simulink model "CIC_decimator_HDL_model"  (R2018b)
settings: Solver=FixedStepAuto  StartTime=0.0  StopTime=10  RelTol=1e-3  EnableMultiTasking=on
values from neighbouring files (symbols this model uses):
  Fs = 2e6    (= 2000000)    [CIC_decimation_with_comp.m]
  ftest1 = 1e3    (= 1000)    [CIC_decimation_with_comp.m]
  ftest2 = 4e3    (= 4000)    [CIC_decimation_with_comp.m]
  ftest3 = 12e3    (= 12000)    [CIC_decimation_with_comp.m]
  hz = int32(round(h * power(2, B - 1) - 1))    [CIC_decimation_with_comp.m]
  R = 125    [CIC_decimation_with_comp.m]
  scaling_numerator = 11    [CIC_decimation_with_comp.m]
undefined symbols (not defined in the file or in its folder): DiscIntNeverNeededParam
libraries: hdlsllib x28, dspsrcs4 x3, simulink x2, commchan3 x1
settings Model: Creator=MrGoshak  LastModifiedBy=MrGoshak
settings HardwareCC: ProdBitPerPointer=32  ProdBitPerSizeT=32  ProdBitPerPtrDiffT=32  ProdLargestAtomicFloat=None  ProdIntDivRoundTo=Undefined  ProdEndianess=Unspecified  ProdWordSize=32  ProdHWDeviceType=ASIC/FPGA->ASIC/FPGA  TargetBitPerPointer=64  TargetBitPerSizeT=64  TargetBitPerPtrDiffT=64  TargetLongLongMode=on  TargetIntDivRoundTo=Zero  TargetEndianess=LittleEndian  TargetWordSize=64  TargetHWDeviceType=Custom Processor->MATLAB Host Computer  ProdEqTarget=off

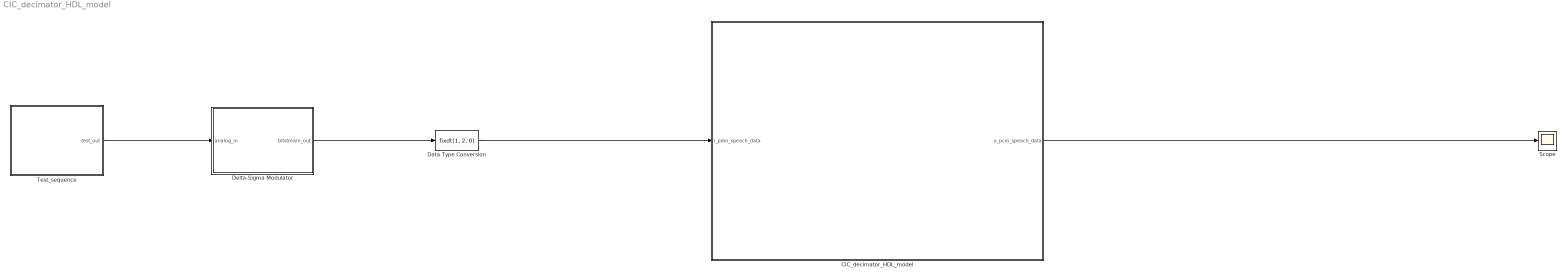
== system CIC_decimator_HDL_model ==
  CIC_decimator_HDL_model : Subsystem
  Data Type Conversion : DataTypeConversion  OutDataTypeStr=fixdt(1, 2, 0)
  "Delta-Sigma Modulator " : Subsystem
  Scope : Scope
  "Test_sequence " : Subsystem
  wires:
  "Test_sequence "/1(test_out) -> "Delta-Sigma Modulator "/1(analog_in)
  "Delta-Sigma Modulator "/1(bitstream_out) -> Data Type Conversion/1
  Data Type Conversion/1 -> CIC_decimator_HDL_model/1(i_pdm_speach_data)
  CIC_decimator_HDL_model/1(o_pcm_speach_data) -> Scope/1

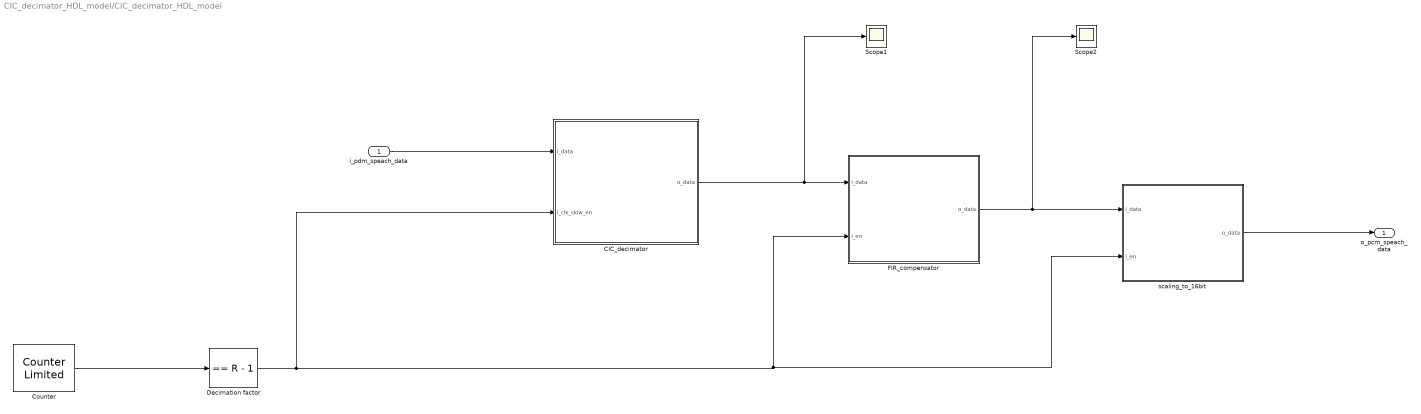
== system CIC_decimator_HDL_model/CIC_decimator_HDL_model ==
  i_pdm_speach_data : Inport
  CIC_decimator : Subsystem  Tag=FilterWizardSubSystem
      settings: ErrorFcn=dspFilterRealizedInBasicElemsAlgLoopErrFcnCallback
  "Counter " : simulink/Sources/Counter Limited  uplimit=R - 1  tsamp=1/Fs
  Decimation factor : simulink/Logic and Bit Operations/Compare To Constant  relop===  const=R - 1  OutDataTypeStr=boolean
  FIR_compensator : Subsystem  Tag=FilterWizardSubSystem
      settings: ErrorFcn=dspFilterRealizedInBasicElemsAlgLoopErrFcnCallback
  Scope1 : Scope
  Scope2 : Scope
  scaling_to_16bit : Subsystem
  o_pcm_speach_data : Outport
  wires:
  FIR_compensator/1(o_data) -> Scope2/1, scaling_to_16bit/1(i_data)
  i_pdm_speach_data/1 -> CIC_decimator/1(i_data)
  CIC_decimator/1(o_data) -> Scope1/1, FIR_compensator/1(i_data)
  scaling_to_16bit/1(o_data) -> o_pcm_speach_data/1
  Decimation factor/1 -> CIC_decimator/2(i_clk_slow_en), FIR_compensator/2(i_en), scaling_to_16bit/2(i_en)
  "Counter "/1 -> Decimation factor/1

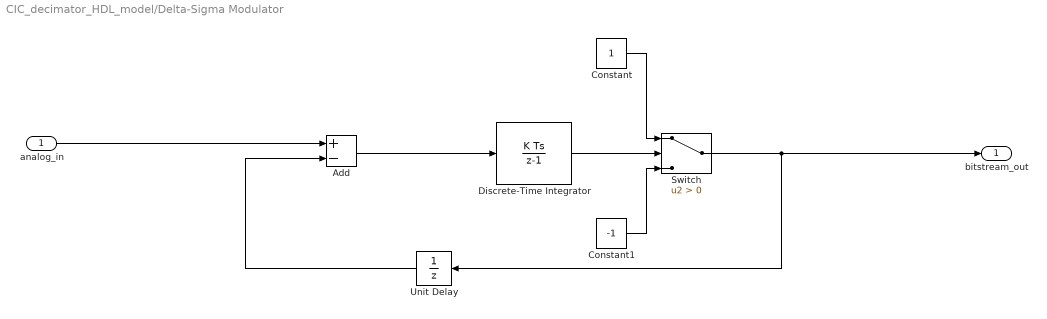
== system CIC_decimator_HDL_model/Delta-Sigma Modulator  ==
  analog_in : Inport
  Add : Sum  Inputs=+-
  Constant : Constant
  Constant1 : Constant  Value=-1
  Discrete-Time Integrator : DiscreteIntegrator  SampleTime=-1  ICPrevOutput=DiscIntNeverNeededParam  ICPrevScaledInput=DiscIntNeverNeededParam
  Switch : Switch  Criteria=u2 > Threshold
  Unit Delay : UnitDelay  SampleTime=-1
  bitstream_out : Outport
  wires:
  Unit Delay/1 -> Add/2
  Discrete-Time Integrator/1 -> Switch/2
  analog_in/1 -> Add/1
  Add/1 -> Discrete-Time Integrator/1
  Constant1/1 -> Switch/3
  Constant/1 -> Switch/1
  Switch/1 -> bitstream_out/1, Unit Delay/1

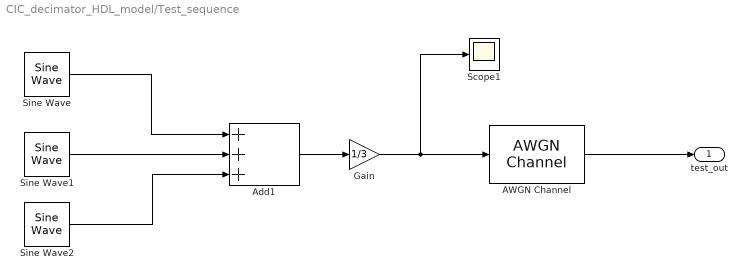
== system CIC_decimator_HDL_model/Test_sequence  ==
  AWGN Channel : commchan3/AWGN Channel  InputProcessing=Columns as channels (frame based)  seed=67  noiseMode="Signal to noise ratio  (SNR)"  EbNodB=10  EsNodB=10  SNRdB=40  bitsPerSym=1  Ps=1  Tsym=1  variance=1
  Add1 : Sum  Inputs=+++
  Gain : Gain  Gain=1/3
  Scope1 : Scope
  Sine Wave : dspsrcs4/Sine Wave  Amplitude=1  Frequency=ftest1  Phase=0  SampleMode=Discrete  OutComplex=Real  CompMethod=Trigonometric fcn  TableSize=Speed  SampleTime=1/Fs  SamplesPerFrame=1  ResetState=Restart at time zero  OutputFrames=off  dataType=double  wordLen=16  udDataType=sfix(16)  fracBitsMode=User-defined  numFracBits=0  OutDataTypeStr=double  LastOutDataTypeStr=double
  Sine Wave1 : dspsrcs4/Sine Wave  Amplitude=1  Frequency=ftest2  Phase=0  SampleMode=Discrete  OutComplex=Real  CompMethod=Trigonometric fcn  TableSize=Speed  SampleTime=1/Fs  SamplesPerFrame=1  ResetState=Restart at time zero  OutputFrames=off  dataType=double  wordLen=16  udDataType=sfix(16)  fracBitsMode=Best precision  numFracBits=15  OutDataTypeStr=double  LastOutDataTypeStr=double
  Sine Wave2 : dspsrcs4/Sine Wave  Amplitude=1  Frequency=ftest3  Phase=0  SampleMode=Discrete  OutComplex=Real  CompMethod=Trigonometric fcn  TableSize=Speed  SampleTime=1/Fs  SamplesPerFrame=1  ResetState=Restart at time zero  OutputFrames=off  dataType=double  wordLen=16  udDataType=sfix(16)  fracBitsMode=Best precision  numFracBits=15  OutDataTypeStr=double  LastOutDataTypeStr=double
  test_out : Outport
  wires:
  Sine Wave2/1 -> Add1/3
  Sine Wave/1 -> Add1/1
  Add1/1 -> Gain/1
  Gain/1 -> AWGN Channel/1, Scope1/1
  Sine Wave1/1 -> Add1/2
  AWGN Channel/1 -> test_out/1

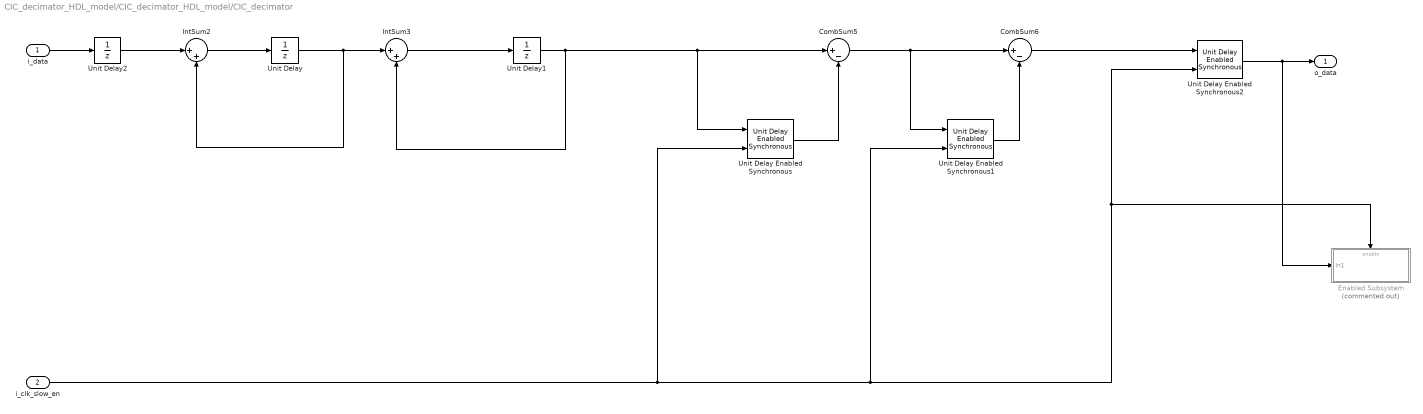
== system CIC_decimator_HDL_model/CIC_decimator_HDL_model/CIC_decimator ==
  i_data : Inport  SampleTime=1/Fs
  i_clk_slow_en : Inport  Port=2
  CombSum5 : Sum  Inputs=|+-  OutDataTypeStr=CIC_data_type
  CombSum6 : Sum  Inputs=|+-  OutDataTypeStr=CIC_data_type
  Enabled Subsystem : Subsystem  Commented=on  TreatAsAtomicUnit=on
  IntSum2 : Sum  Inputs=|++  OutDataTypeStr=CIC_data_type
  IntSum3 : Sum  Inputs=|++  OutDataTypeStr=CIC_data_type
  Unit Delay : UnitDelay  SampleTime=-1
  Unit Delay Enabled Synchronous : hdlsllib/Discrete/Unit Delay Enabled Synchronous  InitialCondition=0.0  SampleTime=-1
      settings: SourceProductName=HDL Coder  SourceProductBaseCode=HD
  Unit Delay Enabled Synchronous1 : hdlsllib/Discrete/Unit Delay Enabled Synchronous  InitialCondition=0.0  SampleTime=-1
      settings: SourceProductName=HDL Coder  SourceProductBaseCode=HD
  Unit Delay Enabled Synchronous2 : hdlsllib/Discrete/Unit Delay Enabled Synchronous  InitialCondition=0.0  SampleTime=-1
      settings: SourceProductName=HDL Coder  SourceProductBaseCode=HD
  Unit Delay1 : UnitDelay  SampleTime=-1
  Unit Delay2 : UnitDelay  SampleTime=-1
  o_data : Outport
  wires:
  i_data/1 -> Unit Delay2/1
  Unit Delay/1 -> IntSum2/2, IntSum3/1
  IntSum3/1 -> Unit Delay1/1
  CombSum5/1 -> Unit Delay Enabled Synchronous1/1, CombSum6/1
  Unit Delay Enabled Synchronous/1 -> CombSum5/2
  Unit Delay Enabled Synchronous1/1 -> CombSum6/2
  CombSum6/1 -> Unit Delay Enabled Synchronous2/1
  Unit Delay Enabled Synchronous2/1 -> Enabled Subsystem/1(In1), o_data/1
  IntSum2/1 -> Unit Delay/1
  Unit Delay1/1 -> IntSum3/2, Unit Delay Enabled Synchronous/1, CombSum5/1
  i_clk_slow_en/1 -> Unit Delay Enabled Synchronous1/2, Enabled Subsystem/Enable, Unit Delay Enabled Synchronous2/2, Unit Delay Enabled Synchronous/2
  Unit Delay2/1 -> IntSum2/1

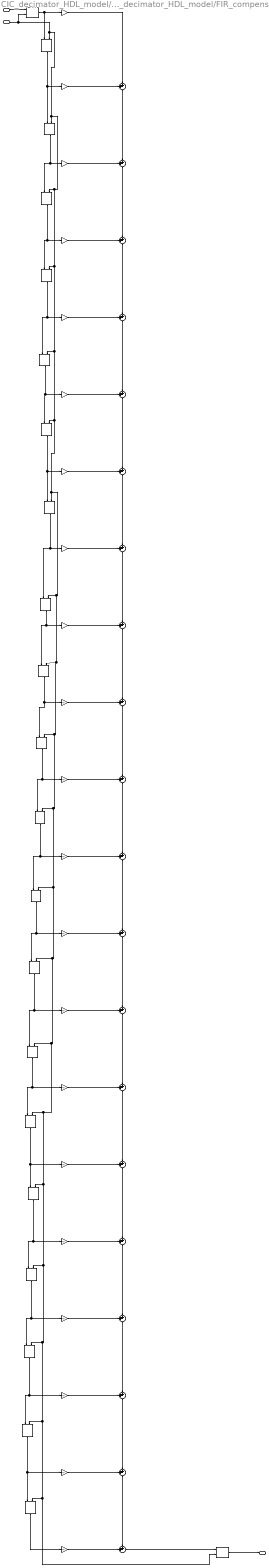
== system CIC_decimator_HDL_model/CIC_decimator_HDL_model/FIR_compensator ==
  i_data : Inport
  i_en : Inport  Port=2
  BodyLSum{2..21} (20 alike) : Sum  Inputs=++|  AccumDataTypeStr=FIR_product_data_type  OutDataTypeStr=FIR_product_data_type  SaturateOnIntegerOverflow=on
  Unit Delay Enabled Synchronous{,1..21} (22 alike) : hdlsllib/Discrete/Unit Delay Enabled Synchronous  InitialCondition=0.0  SampleTime=-1
      settings: SourceProductName=HDL Coder  SourceProductBaseCode=HD
  b(1) : Gain  Gain=hz(1)  ParamDataTypeStr=FIR_coeffs_data_type  OutDataTypeStr=FIR_product_data_type  SaturateOnIntegerOverflow=on
  b(10) : Gain  Gain=hz(10)  ParamDataTypeStr=FIR_coeffs_data_type  OutDataTypeStr=FIR_product_data_type  SaturateOnIntegerOverflow=on
  b(11) : Gain  Gain=hz(11)  ParamDataTypeStr=FIR_coeffs_data_type  OutDataTypeStr=FIR_product_data_type  SaturateOnIntegerOverflow=on
  b(12) : Gain  Gain=hz(12)  ParamDataTypeStr=FIR_coeffs_data_type  OutDataTypeStr=FIR_product_data_type  SaturateOnIntegerOverflow=on
  b(13) : Gain  Gain=hz(13)  ParamDataTypeStr=FIR_coeffs_data_type  OutDataTypeStr=FIR_product_data_type  SaturateOnIntegerOverflow=on
  b(14) : Gain  Gain=hz(14)  ParamDataTypeStr=FIR_coeffs_data_type  OutDataTypeStr=FIR_product_data_type  SaturateOnIntegerOverflow=on
  b(15) : Gain  Gain=hz(15)  ParamDataTypeStr=FIR_coeffs_data_type  OutDataTypeStr=FIR_product_data_type  SaturateOnIntegerOverflow=on
  b(16) : Gain  Gain=hz(16)  ParamDataTypeStr=FIR_coeffs_data_type  OutDataTypeStr=FIR_product_data_type  SaturateOnIntegerOverflow=on
  b(17) : Gain  Gain=hz(17)  ParamDataTypeStr=FIR_coeffs_data_type  OutDataTypeStr=FIR_product_data_type  SaturateOnIntegerOverflow=on
  b(18) : Gain  Gain=hz(18)  ParamDataTypeStr=FIR_coeffs_data_type  OutDataTypeStr=FIR_product_data_type  SaturateOnIntegerOverflow=on
  b(19) : Gain  Gain=hz(19)  ParamDataTypeStr=FIR_coeffs_data_type  OutDataTypeStr=FIR_product_data_type  SaturateOnIntegerOverflow=on
  b(2) : Gain  Gain=hz(2)  ParamDataTypeStr=FIR_coeffs_data_type  OutDataTypeStr=FIR_product_data_type  SaturateOnIntegerOverflow=on
  b(20) : Gain  Gain=hz(20)  ParamDataTypeStr=FIR_coeffs_data_type  OutDataTypeStr=FIR_product_data_type  SaturateOnIntegerOverflow=on
  b(21) : Gain  Gain=hz(21)  ParamDataTypeStr=FIR_coeffs_data_type  OutDataTypeStr=FIR_product_data_type  SaturateOnIntegerOverflow=on
  b(3) : Gain  Gain=hz(3)  ParamDataTypeStr=FIR_coeffs_data_type  OutDataTypeStr=FIR_product_data_type  SaturateOnIntegerOverflow=on
  b(4) : Gain  Gain=hz(4)  ParamDataTypeStr=FIR_coeffs_data_type  OutDataTypeStr=FIR_product_data_type  SaturateOnIntegerOverflow=on
  b(5) : Gain  Gain=hz(5)  ParamDataTypeStr=FIR_coeffs_data_type  OutDataTypeStr=FIR_product_data_type  SaturateOnIntegerOverflow=on
  b(6) : Gain  Gain=hz(6)  ParamDataTypeStr=FIR_coeffs_data_type  OutDataTypeStr=FIR_product_data_type  SaturateOnIntegerOverflow=on
  b(7) : Gain  Gain=hz(7)  ParamDataTypeStr=FIR_coeffs_data_type  OutDataTypeStr=FIR_product_data_type  SaturateOnIntegerOverflow=on
  b(8) : Gain  Gain=hz(8)  ParamDataTypeStr=FIR_coeffs_data_type  OutDataTypeStr=FIR_product_data_type  SaturateOnIntegerOverflow=on
  b(9) : Gain  Gain=hz(9)  ParamDataTypeStr=FIR_coeffs_data_type  OutDataTypeStr=FIR_product_data_type  SaturateOnIntegerOverflow=on
  o_data : Outport
  wires:
  b(1)/1 -> BodyLSum2/2
  Unit Delay Enabled Synchronous/1 -> Unit Delay Enabled Synchronous1/1, b(2)/1
  b(2)/1 -> BodyLSum2/1
  BodyLSum2/1 -> BodyLSum3/2
  b(3)/1 -> BodyLSum3/1
  BodyLSum3/1 -> BodyLSum4/2
  Unit Delay Enabled Synchronous2/1 -> Unit Delay Enabled Synchronous3/1, b(4)/1
  b(4)/1 -> BodyLSum4/1
  BodyLSum4/1 -> BodyLSum5/2
  Unit Delay Enabled Synchronous3/1 -> b(5)/1, Unit Delay Enabled Synchronous4/1
  b(5)/1 -> BodyLSum5/1
  BodyLSum5/1 -> BodyLSum6/2
  b(6)/1 -> BodyLSum6/1
  BodyLSum6/1 -> BodyLSum7/2
  Unit Delay Enabled Synchronous5/1 -> b(7)/1, Unit Delay Enabled Synchronous6/1
  b(7)/1 -> BodyLSum7/1
  BodyLSum7/1 -> BodyLSum8/2
  b(8)/1 -> BodyLSum8/1
  BodyLSum8/1 -> BodyLSum9/2
  b(9)/1 -> BodyLSum9/1
  BodyLSum9/1 -> BodyLSum10/2
  b(10)/1 -> BodyLSum10/1
  BodyLSum10/1 -> BodyLSum11/2
  b(11)/1 -> BodyLSum11/1
  BodyLSum11/1 -> BodyLSum12/2
  b(12)/1 -> BodyLSum12/1
  BodyLSum12/1 -> BodyLSum13/2
  b(13)/1 -> BodyLSum13/1
  BodyLSum13/1 -> BodyLSum14/2
  b(14)/1 -> BodyLSum14/1
  BodyLSum14/1 -> BodyLSum15/2
  b(15)/1 -> BodyLSum15/1
  BodyLSum15/1 -> BodyLSum16/2
  b(16)/1 -> BodyLSum16/1
  BodyLSum16/1 -> BodyLSum17/2
  b(17)/1 -> BodyLSum17/1
  BodyLSum17/1 -> BodyLSum18/2
  b(18)/1 -> BodyLSum18/1
  BodyLSum18/1 -> BodyLSum19/2
  b(19)/1 -> BodyLSum19/1
  BodyLSum19/1 -> BodyLSum20/2
  b(20)/1 -> BodyLSum20/1
  BodyLSum20/1 -> BodyLSum21/1
  b(21)/1 -> BodyLSum21/2
  Unit Delay Enabled Synchronous1/1 -> Unit Delay Enabled Synchronous2/1, b(3)/1
  Unit Delay Enabled Synchronous4/1 -> b(6)/1, Unit Delay Enabled Synchronous5/1
  Unit Delay Enabled Synchronous6/1 -> Unit Delay Enabled Synchronous7/1, b(8)/1
  Unit Delay Enabled Synchronous7/1 -> Unit Delay Enabled Synchronous8/1, b(9)/1
  Unit Delay Enabled Synchronous8/1 -> Unit Delay Enabled Synchronous9/1, b(10)/1
  Unit Delay Enabled Synchronous9/1 -> Unit Delay Enabled Synchronous10/1, b(11)/1
  Unit Delay Enabled Synchronous10/1 -> Unit Delay Enabled Synchronous11/1, b(12)/1
  Unit Delay Enabled Synchronous11/1 -> Unit Delay Enabled Synchronous12/1, b(13)/1
  Unit Delay Enabled Synchronous12/1 -> Unit Delay Enabled Synchronous13/1, b(14)/1
  Unit Delay Enabled Synchronous13/1 -> Unit Delay Enabled Synchronous14/1, b(15)/1
  Unit Delay Enabled Synchronous14/1 -> b(16)/1, Unit Delay Enabled Synchronous15/1
  Unit Delay Enabled Synchronous15/1 -> Unit Delay Enabled Synchronous16/1, b(17)/1
  Unit Delay Enabled Synchronous16/1 -> Unit Delay Enabled Synchronous17/1, b(18)/1
  Unit Delay Enabled Synchronous17/1 -> b(19)/1, Unit Delay Enabled Synchronous18/1
  Unit Delay Enabled Synchronous18/1 -> b(20)/1, Unit Delay Enabled Synchronous19/1
  Unit Delay Enabled Synchronous19/1 -> b(21)/1
  Unit Delay Enabled Synchronous20/1 -> o_data/1
  i_data/1 -> Unit Delay Enabled Synchronous21/1
  Unit Delay Enabled Synchronous21/1 -> Unit Delay Enabled Synchronous/1, b(1)/1
  i_en/1 -> Unit Delay Enabled Synchronous20/2, Unit Delay Enabled Synchronous19/2, Unit Delay Enabled Synchronous18/2, Unit Delay Enabled Synchronous17/2, Unit Delay Enabled Synchronous16/2, Unit Delay Enabled Synchronous15/2, Unit Delay Enabled Synchronous14/2, Unit Delay Enabled Synchronous13/2, Unit Delay Enabled Synchronous12/2, Unit Delay Enabled Synchronous11/2, Unit Delay Enabled Synchronous10/2, Unit Delay Enabled Synchronous9/2, Unit Delay Enabled Synchronous8/2, Unit Delay Enabled Synchronous7/2, Unit Delay Enabled Synchronous6/2, Unit Delay Enabled Synchronous5/2, Unit Delay Enabled Synchronous4/2, Unit Delay Enabled Synchronous3/2, Unit Delay Enabled Synchronous2/2, Unit Delay Enabled Synchronous1/2, Unit Delay Enabled Synchronous/2, Unit Delay Enabled Synchronous21/2
  BodyLSum21/1 -> Unit Delay Enabled Synchronous20/1

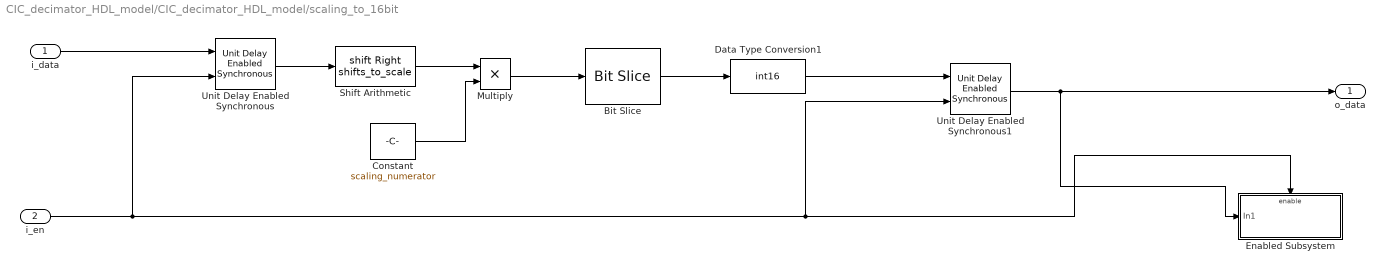
== system CIC_decimator_HDL_model/CIC_decimator_HDL_model/scaling_to_16bit ==
  i_data : Inport
  i_en : Inport  Port=2
  Bit Slice : hdlsllib/Logic and Bit Operations/Bit Slice  lidx=30  ridx=15
  Constant : Constant  Value=scaling_numerator  OutDataTypeStr=uint8  SampleTime=1/Fs
  Data Type Conversion1 : DataTypeConversion  OutDataTypeStr=int16
  Enabled Subsystem : Subsystem  TreatAsAtomicUnit=on
  Multiply : Product  OutDataTypeStr=fixdt(1,31,0)  SaturateOnIntegerOverflow=on
  Shift Arithmetic : ArithShift  BitShiftNumber=shifts_to_scale  BitShiftDirection=Right
  Unit Delay Enabled Synchronous : hdlsllib/Discrete/Unit Delay Enabled Synchronous  InitialCondition=0.0  SampleTime=-1
      settings: SourceProductName=HDL Coder  SourceProductBaseCode=HD
  Unit Delay Enabled Synchronous1 : hdlsllib/Discrete/Unit Delay Enabled Synchronous  InitialCondition=0.0  SampleTime=-1
      settings: SourceProductName=HDL Coder  SourceProductBaseCode=HD
  o_data : Outport
  wires:
  Bit Slice/1 -> Data Type Conversion1/1
  Constant/1 -> Multiply/2
  Shift Arithmetic/1 -> Multiply/1
  Multiply/1 -> Bit Slice/1
  Unit Delay Enabled Synchronous/1 -> Shift Arithmetic/1
  i_data/1 -> Unit Delay Enabled Synchronous/1
  Data Type Conversion1/1 -> Unit Delay Enabled Synchronous1/1
  Unit Delay Enabled Synchronous1/1 -> Enabled Subsystem/1(In1), o_data/1
  i_en/1 -> Unit Delay Enabled Synchronous/2, Unit Delay Enabled Synchronous1/2, Enabled Subsystem/Enable

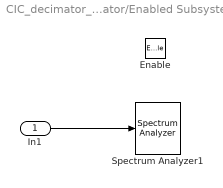
== system CIC_decimator_HDL_model/CIC_decimator_HDL_model/CIC_decimator/Enabled Subsystem ==
  In1 : Inport
  Enable : EnablePort
  Spectrum Analyzer1 : SpectrumAnalyzer
  wires:
  In1/1 -> Spectrum Analyzer1/1

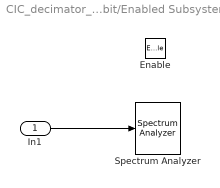
== system CIC_decimator_HDL_model/CIC_decimator_HDL_model/scaling_to_16bit/Enabled Subsystem ==
  In1 : Inport
  Enable : EnablePort
  Spectrum Analyzer : SpectrumAnalyzer
  wires:
  In1/1 -> Spectrum Analyzer/1
